simulink model "dc_motor_5hp_model1"  (R2017b)
settings: Solver=ode45  StartTime=0.0  StopTime=6  RelTol=1e-3  EnableMultiTasking=on
undefined symbols (not defined in the file): Dm, J, Laf, Ra, Rf, Ta, Tf, Tm, Va
settings Model: Creator=Jurij  LastModifiedBy=Jurij
settings DataIOCC: LimitDataPoints=on  MaxDataPoints=10000  SaveFormat=Array  SignalLoggingSaveFormat=ModelDataLogs  SaveOutput=off  SaveState=on  StateSaveName=x  TimeSaveName=t  SignalLoggingName=sigsOut
settings OptimizationCC: LifeSpan=inf
settings DebuggingCC: SaveWithParameterizedLinksMsg=none  UnderspecifiedInitializationDetection=Classic  MergeDetectMultiDrivingBlocksExec=none  SignalResolutionControl=TryResolveAllWithWarning  MultiTaskDSMMsg=warning  MultiTaskCondExecSysMsg=none  SFUnexpectedBacktrackingDiag=warning  SFNoUnconditionalDefaultTransitionDiag=warning  SFExecutionAtInitializationDiag=none
settings HardwareCC: ProdBitPerPointer=32  ProdBitPerSizeT=32  ProdBitPerPtrDiffT=32  ProdLargestAtomicFloat=None  ProdIntDivRoundTo=Undefined  ProdEndianess=Unspecified  ProdWordSize=32  ProdHWDeviceType=32-bit Generic  TargetUnknown=on
settings ModelReferenceCC: PropagateSignalLabelsOutOfModel=off
settings CodeAppCC: StateflowObjectComments=on
settings GRTTargetCC: TargetLangStandard=C89/C90 (ANSI)  GeneratePreprocessorConditionals=Disable all  CombineOutputUpdateFcns=off  GRTInterface=on
settings ConfigComp: CovMetricSettings=dw  CovHtmlReporting=on  CovSaveCumulativeToWorkspaceVar=on  CovSaveSingleToWorkspaceVar=on  CovExternalEMLEnable=off

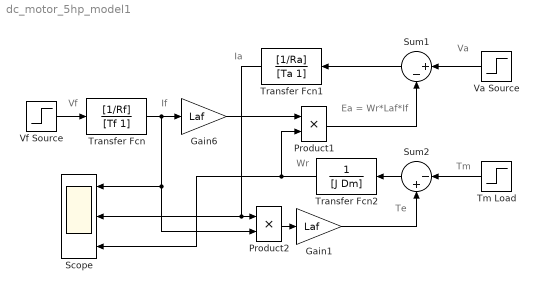
== system dc_motor_5hp_model1 ==
  note: Ia
  note: If
  note: Ea = Wr*Laf*If
  note: Wr
  note: Te
  note: Tm
  note: Va
  note: Vf
  Gain1 : Gain  Gain=Laf  SaturateOnIntegerOverflow=on  OutDataTypeStr=Inherit: Same as input  ParamDataTypeStr=Inherit: Same as input
  Gain6 : Gain  Gain=Laf  SaturateOnIntegerOverflow=on  OutDataTypeStr=Inherit: Same as input  ParamDataTypeStr=Inherit: Same as input
  Product1 : Product  SaturateOnIntegerOverflow=on  OutDataTypeStr=Inherit: Same as first input
  Product2 : Product  SaturateOnIntegerOverflow=on  OutDataTypeStr=Inherit: Same as first input
  Scope : Scope  NumInputPorts=3
  Sum1 : Sum  Inputs=|+-  SaturateOnIntegerOverflow=on
  Sum2 : Sum  Inputs=|-+  SaturateOnIntegerOverflow=on
  Tm Load : Step  Time=4  After=Tm  SampleTime=0
  Transfer Fcn : TransferFcn  Numerator=[1/Rf]  Denominator=[Tf 1]
  Transfer Fcn1 : TransferFcn  Numerator=[1/Ra]  Denominator=[Ta 1]
  Transfer Fcn2 : TransferFcn  Denominator=[J Dm]
  Va Source : Step  Time=2  After=Va  SampleTime=0
  Vf Source : Step  Time=0  Before=Va  After=Va  SampleTime=0
  wires:
  Transfer Fcn/1 -> Gain6/1, Product2/2, Scope/1
  Gain6/1 -> Product1/1
  Sum1/1 -> Transfer Fcn1/1
  Va Source/1 -> Sum1/1
  Vf Source/1 -> Transfer Fcn/1
  Transfer Fcn2/1 -> Product1/2, Scope/3
  Product1/1 -> Sum1/2
  Sum2/1 -> Transfer Fcn2/1
  Tm Load/1 -> Sum2/1
  Product2/1 -> Gain1/1
  Transfer Fcn1/1 -> Product2/1, Scope/2
  Gain1/1 -> Sum2/2
